simulink model "aircraft_6dof"  (R2025a)
settings: Solver=VariableStepAuto  StartTime=0.0  StopTime=sim_params.duration  FixedStep=0.01  RelTol=1e-8
undefined symbols (not defined in the file): aero, aircraft, atmos, control, controller, engine, IC
libraries: aerolibactuator x5, aerolibasang x2, aerolibfltsims x2, aerolibtransform2 x1, aerolibatmos2 x1, aerolibanimutils x1
settings Model: Creator=lordf  LastModifiedBy=lordf
settings DataIOCC: ExternalInput=getinputstruct(report1)  InitialState=getstatestruct(report1)

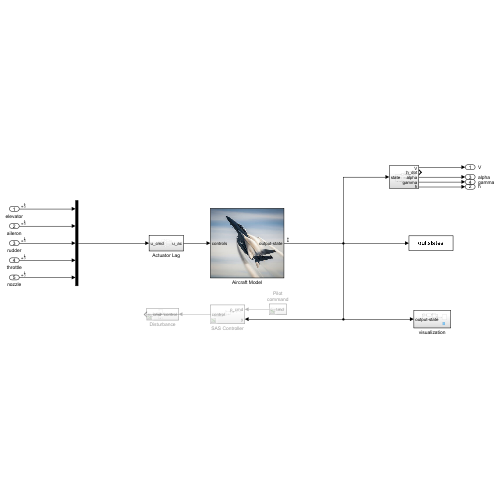
[thumbnail: Simulink's stored preview of the top-level diagram]
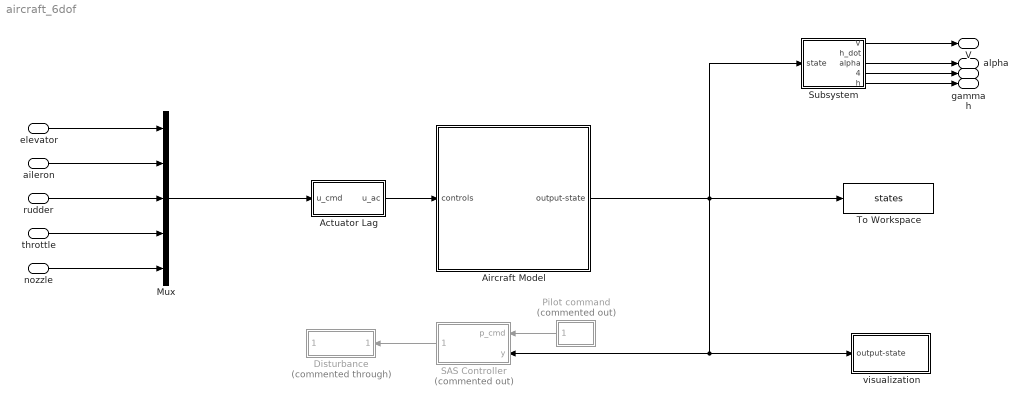
== system aircraft_6dof ==
  elevator : Inport
  aileron : Inport  Port=2
  rudder : Inport  Port=3
  throttle : Inport  Port=4
  nozzle : Inport  Port=5
  Actuator Lag : Subsystem
  Aircraft Model : Subsystem
      mask Display: image('Aircraft_image.jpg');
  Disturbance : Subsystem  Commented=through
  Mux : Mux  Inputs=5
  Pilot command : Subsystem  Commented=on
  SAS Controller : Subsystem  Commented=on
  Subsystem : Subsystem
  To Workspace : ToWorkspace  VariableName=states  SampleTime=-1
  visualization : Subsystem
  V : Outport
  h : Outport  Port=2
  alpha : Outport  Port=3
  gamma : Outport  Port=4
  wires:
  Subsystem/5(h) -> h/1
  Subsystem/1(V) -> V/1
  Subsystem/4(gamma) -> gamma/1
  Subsystem/3(alpha) -> alpha/1
  Actuator Lag/1(u_ac) -> Aircraft Model/1(controls)
  SAS Controller/1(control) -> Disturbance/1(control)
  Pilot command/1(p_cmd) -> SAS Controller/1(p_cmd)
  Aircraft Model/1(output-state) -> SAS Controller/2(y), visualization/1(output-state), Subsystem/1(state), To Workspace/1
  nozzle/1 -> Mux/5
  throttle/1 -> Mux/4
  aileron/1 -> Mux/2
  rudder/1 -> Mux/3
  elevator/1 -> Mux/1
  Mux/1 -> Actuator Lag/1(u_cmd)

== system aircraft_6dof/Actuator Lag ==
  u_cmd : Inport
  Demux : Demux  Outputs=5
  Mux : Mux  Inputs=5
  aileron lag : Subsystem
  elevator lag : Subsystem
  nozzle lag : Subsystem
  rudder lag : Subsystem
  throttle lag : Subsystem
  u_ac : Outport
  wires:
  u_cmd/1 -> Demux/1
  Mux/1 -> u_ac/1
  Demux/1 -> elevator lag/1(In1)
  elevator lag/1(Out1) -> Mux/1
  Demux/2 -> aileron lag/1(In1)
  aileron lag/1(Out1) -> Mux/2
  Demux/3 -> rudder lag/1(In1)
  rudder lag/1(Out1) -> Mux/3
  Demux/4 -> throttle lag/1(In1)
  throttle lag/1(Out1) -> Mux/4
  Demux/5 -> nozzle lag/1(In1)
  nozzle lag/1(Out1) -> Mux/5

== system aircraft_6dof/Aircraft Model ==
  controls : Inport
  6DOF (Euler Angles) : EOM6DOFBodyEuler  xme_0=[IC.x IC.y IC.z]  Vm_0=[IC.u, IC.v, IC.w]  eul_0=[IC.phi IC.theta IC.psi]  pm_0=[IC.p IC.q IC.r]  mass_0=aircraft.mass  inertia=aircraft.I
  Forces and Moments : Subsystem
  Mux1 : Mux
  output-state : Outport
  wires:
  6DOF (Euler Angles)/3 -> Mux1/4  "attitude(earth)"
  6DOF (Euler Angles)/5 -> Mux1/1  "velocity(body)"
  Forces and Moments/2(M) -> 6DOF (Euler Angles)/2
  6DOF (Euler Angles)/2 -> Mux1/2  "Position(earth)"
  Forces and Moments/1(F) -> 6DOF (Euler Angles)/1
  6DOF (Euler Angles)/6 -> Mux1/3  "omega(body)"
  controls/1 -> Forces and Moments/2(controls)
  Mux1/1 -> Forces and Moments/1(state), output-state/1

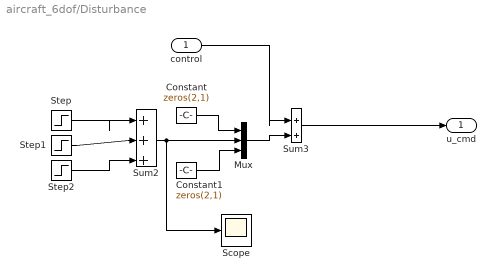
== system aircraft_6dof/Disturbance ==
  control : Inport
  Constant : Constant  Value=zeros(2,1)
  Constant1 : Constant  Value=zeros(2,1)
  Mux : Mux  Inputs=3
  Scope : Scope
      settings: ActiveDisplayYMinimum=-0.125  ActiveDisplayYMaximum=0.125
  Step : Step  Time=10  After=0.1  SampleTime=0
  Step1 : Step  Time=11  After=-0.2  SampleTime=0
  Step2 : Step  Time=12  After=0.1  SampleTime=0
  Sum2 : Sum  Inputs=|+++
  Sum3 : Sum  Inputs=|++
  u_cmd : Outport
  wires:
  Sum2/1 -> Mux/2, Scope/1
  Step/1 -> Sum2/1
  Step2/1 -> Sum2/3
  Step1/1 -> Sum2/2
  Sum3/1 -> u_cmd/1
  control/1 -> Sum3/1
  Mux/1 -> Sum3/2
  Constant/1 -> Mux/1
  Constant1/1 -> Mux/3

== system aircraft_6dof/Pilot command ==
  Gain : Gain  Gain=0.4
  Mux : Mux  Inputs=3
  Pilot Joystick : aerolibanimutils/Pilot Joystick  JoystickID=Joystick1  OutputConfiguration=FourAxis  SampleTime=1/30
  p_cmd : Outport
  wires:
  Mux/1 -> Gain/1
  Pilot Joystick/1 -> Mux/1
  Pilot Joystick/2 -> Mux/2
  Pilot Joystick/3 -> Mux/3
  Gain/1 -> p_cmd/1

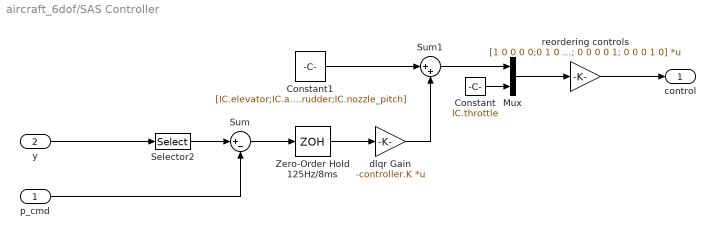
== system aircraft_6dof/SAS Controller ==
  p_cmd : Inport
  y : Inport  Port=2
  Constant : Constant  Value=IC.throttle
  Constant1 : Constant  Value=[IC.elevator;IC.aileron;IC.rudder;IC.nozzle_pitch]
  Mux : Mux  Inputs=2
  Selector2 : Selector  InputPortWidth=12  IndexOptions=Index vector (dialog)  Indices=7:9  OutputSizes=1
  Sum : Sum  Inputs=|+-
  Sum1 : Sum  Inputs=|++
  Zero-Order Hold 125Hz/8ms : ZeroOrderHold  SampleTime=controller.Ts
  dlqr Gain : Gain  Gain=-controller.K  Multiplication=Matrix(K*u)
  reordering controls : Gain  Gain=[1 0 0 0 0;0 1 0 0 0;0 0 1 0 0; 0 0 0 0 1; 0 0 0 1 0]  Multiplication=Matrix(K*u)
  control : Outport
  wires:
  Selector2/1 -> Sum/1
  y/1 -> Selector2/1
  Mux/1 -> reordering controls/1
  Constant1/1 -> Sum1/1
  Constant/1 -> Mux/2
  reordering controls/1 -> control/1
  Sum1/1 -> Mux/1
  dlqr Gain/1 -> Sum1/2
  Sum/1 -> Zero-Order Hold 125Hz/8ms/1
  p_cmd/1 -> Sum/2
  Zero-Order Hold 125Hz/8ms/1 -> dlqr Gain/1

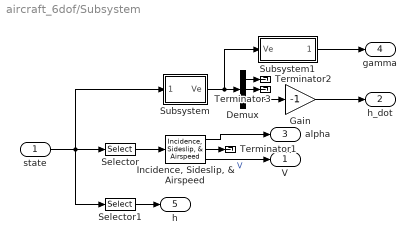
== system aircraft_6dof/Subsystem ==
  state : Inport
  Demux : Demux  Outputs=3
  Gain : Gain  Gain=-1
  "Incidence, Sideslip, & Airspeed" : aerolibasang/Incidence, Sideslip, & Airspeed
  Selector : Selector  InputPortWidth=12  IndexOptions=Index vector (dialog)  Indices=1:3  OutputSizes=1
  Selector1 : Selector  InputPortWidth=12  IndexOptions=Index vector (dialog)  Indices=6  OutputSizes=1
  Subsystem : Subsystem
  Subsystem1 : Subsystem
  Terminator1 : Terminator
  Terminator2 : Terminator
  Terminator3 : Terminator
  V : Outport
  h_dot : Outport  Port=2
  alpha : Outport  Port=3
  gamma : Outport  Port=4
  h : Outport  Port=5
  wires:
  Selector/1 -> "Incidence, Sideslip, & Airspeed"/1
  "Incidence, Sideslip, & Airspeed"/1 -> alpha/1
  "Incidence, Sideslip, & Airspeed"/2 -> Terminator1/1
  "Incidence, Sideslip, & Airspeed"/3 -> V/1  "V"
  Selector1/1 -> h/1
  state/1 -> Subsystem/1(state), Selector1/1, Selector/1
  Subsystem/1(Ve) -> Subsystem1/1(Ve), Demux/1
  Demux/3 -> Gain/1
  Demux/1 -> Terminator2/1
  Demux/2 -> Terminator3/1
  Gain/1 -> h_dot/1
  Subsystem1/1(gamma) -> gamma/1

== system aircraft_6dof/visualization ==
  output-state : Inport
  Constant : Constant  Value=-100
  Demux : Demux  Outputs=2
  Flat Earth to LLA : FlatEarth2LLA  LL0=[37.6655 -122.4809]
  FlightGear Preconfigured 6DoF Animation : aerolibfltsims/FlightGear Preconfigured 6DoF Animation  xFlightGearVersion=v2019.1  DestinationIpAddress=127.0.0.1  DestinationPort=5502  SampleTime=1/30  packetVersion=24
  Generate Run Script : aerolibfltsims/Generate Run Script  Architecture=Mac  dataFlow=Send  GeometryModelName=c172p  AirportId=KSFO  RunwayId=10L  InitialAltitude=7224  InitialHeading=113  OffsetDistance=4.72  OffsetAzimuth=0  InstallScenery=off  DisableShaders=off  OriginAddress=127.0.0.1  DestinationPort=5502  OriginPort=5505  LocalAddress=127.0.0.1  OutputFileName=runfg.bat  FlightGearBaseDirectory=C:\Program Files\FlightGear 2024.1
  Mux : Mux
  Selector : Selector  InputPortWidth=12  IndexOptions=Index vector (dialog)  Indices=10:12  OutputSizes=1
  Selector1 : Selector  InputPortWidth=12  IndexOptions=Index vector (dialog)  Indices=4:6  OutputSizes=1
  wires:
  output-state/1 -> Selector1/1, Selector/1
  Mux/1 -> FlightGear Preconfigured 6DoF Animation/1
  Selector/1 -> Mux/4
  Constant/1 -> Flat Earth to LLA/2
  Flat Earth to LLA/1 -> Demux/1
  Flat Earth to LLA/2 -> Mux/3
  Selector1/1 -> Flat Earth to LLA/1
  Demux/1 -> Mux/2
  Demux/2 -> Mux/1

== system aircraft_6dof/Actuator Lag/aileron lag ==
  In1 : Inport
  Linear Second-Order Actuator : aerolibactuator/Linear Second-Order Actuator  wn_fin=control.wn_aileron  z_fin=control.zeta_aileron  fin_act_0=IC.aileron  fin_act_vel=0
  Rate Limiter1 : RateLimiter  RisingSlewLimit=control.max_aileron_rate  FallingSlewLimit=-control.max_aileron_rate  SampleTimeMode=inherited
  Saturation1 : Saturate  UpperLimit=control.aileron_max  LowerLimit=-control.aileron_max
  Out1 : Outport
  wires:
  Linear Second-Order Actuator/1 -> Saturation1/1
  In1/1 -> Rate Limiter1/1
  Rate Limiter1/1 -> Linear Second-Order Actuator/1
  Saturation1/1 -> Out1/1

== system aircraft_6dof/Actuator Lag/elevator lag ==
  In1 : Inport
  Linear Second-Order Actuator : aerolibactuator/Linear Second-Order Actuator  wn_fin=control.wn_elevator  z_fin=control.zeta_elevator  fin_act_0=IC.elevator  fin_act_vel=0
  Rate Limiter : RateLimiter  RisingSlewLimit=control.max_elevator_rate  FallingSlewLimit=-control.max_elevator_rate  SampleTimeMode=inherited
  Saturation : Saturate  UpperLimit=control.elevator_max  LowerLimit=-control.elevator_max
  Out1 : Outport
  wires:
  In1/1 -> Rate Limiter/1
  Saturation/1 -> Out1/1
  Linear Second-Order Actuator/1 -> Saturation/1
  Rate Limiter/1 -> Linear Second-Order Actuator/1

== system aircraft_6dof/Actuator Lag/nozzle lag ==
  In1 : Inport
  Linear Second-Order Actuator : aerolibactuator/Linear Second-Order Actuator  wn_fin=control.wn_nozzle  z_fin=control.zeta_nozzle  fin_act_0=IC.nozzle_pitch  fin_act_vel=0
  Rate Limiter4 : RateLimiter  RisingSlewLimit=control.max_nozzle_rate  FallingSlewLimit=-control.max_nozzle_rate  SampleTimeMode=inherited
  Saturation4 : Saturate  UpperLimit=control.nozzle_pitch_max  LowerLimit=-control.nozzle_pitch_max
  Out1 : Outport
  wires:
  Rate Limiter4/1 -> Linear Second-Order Actuator/1
  Linear Second-Order Actuator/1 -> Saturation4/1
  Saturation4/1 -> Out1/1
  In1/1 -> Rate Limiter4/1

== system aircraft_6dof/Actuator Lag/rudder lag ==
  In1 : Inport
  Linear Second-Order Actuator : aerolibactuator/Linear Second-Order Actuator  wn_fin=control.wn_rudder  z_fin=control.zeta_rudder  fin_act_0=IC.rudder  fin_act_vel=0
  Rate Limiter2 : RateLimiter  RisingSlewLimit=control.max_rudder_rate  FallingSlewLimit=-control.max_rudder_rate  SampleTimeMode=inherited
  Saturation2 : Saturate  UpperLimit=control.rudder_max  LowerLimit=-control.rudder_max
  Out1 : Outport
  wires:
  Rate Limiter2/1 -> Linear Second-Order Actuator/1
  Linear Second-Order Actuator/1 -> Saturation2/1
  Saturation2/1 -> Out1/1
  In1/1 -> Rate Limiter2/1

== system aircraft_6dof/Actuator Lag/throttle lag ==
  In1 : Inport
  Linear Second-Order Actuator : aerolibactuator/Linear Second-Order Actuator  wn_fin=control.wn_throttle  z_fin=control.zeta_throttle  fin_act_0=IC.throttle  fin_act_vel=0
  Rate Limiter3 : RateLimiter  RisingSlewLimit=control.max_throttle_rate  FallingSlewLimit=-control.max_throttle_rate  SampleTimeMode=inherited
  Saturation3 : Saturate  UpperLimit=1  LowerLimit=0
  Out1 : Outport
  wires:
  Rate Limiter3/1 -> Linear Second-Order Actuator/1
  Saturation3/1 -> Out1/1
  Linear Second-Order Actuator/1 -> Saturation3/1
  In1/1 -> Rate Limiter3/1

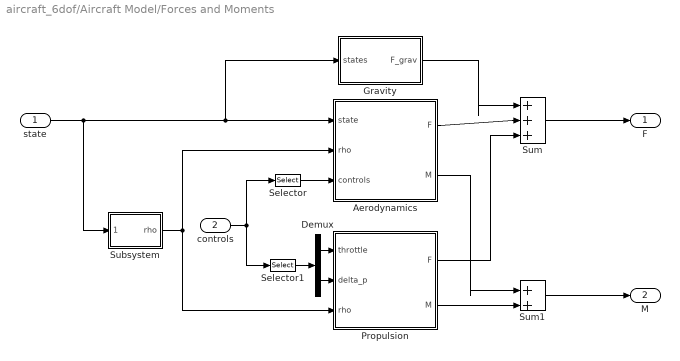
== system aircraft_6dof/Aircraft Model/Forces and Moments ==
  state : Inport
  controls : Inport  Port=2
  Aerodynamics : Subsystem
  Demux : Demux  Outputs=2
  Gravity : Subsystem
  Propulsion : Subsystem
  Selector : Selector  InputPortWidth=5  IndexOptions=Index vector (dialog)  Indices=1:3  OutputSizes=1
  Selector1 : Selector  InputPortWidth=5  IndexOptions=Index vector (dialog)  Indices=4:5  OutputSizes=1
  Subsystem : Subsystem
  Sum : Sum  Inputs=|+++
  Sum1 : Sum  Inputs=|++
  F : Outport
  M : Outport  Port=2
  wires:
  Sum/1 -> F/1
  Aerodynamics/1(F) -> Sum/2
  Aerodynamics/2(M) -> Sum1/1
  Gravity/1(F_grav) -> Sum/1
  Sum1/1 -> M/1
  Demux/1 -> Propulsion/1(throttle)
  Demux/2 -> Propulsion/2(delta_p)
  Propulsion/1(F) -> Sum/3
  Propulsion/2(M) -> Sum1/2
  Subsystem/1(rho) -> Aerodynamics/2(rho), Propulsion/3(rho)
  Selector/1 -> Aerodynamics/3(controls)
  Selector1/1 -> Demux/1
  controls/1 -> Selector1/1, Selector/1
  state/1 -> Subsystem/1(states), Aerodynamics/1(state), Gravity/1(states)

== system aircraft_6dof/Subsystem/Subsystem ==
  state : Inport
  Matrix Multiply : Product  Multiplication=Matrix(*)
  Rotation Angles to Direction Cosine Matrix : Angle2Dcm
      settings: AttributesFormatString=Rotation Order: %<rotationOrder>
  Selector : Selector  InputPortWidth=12  IndexOptions=Index vector (dialog)  Indices=10:12  OutputSizes=1
  Selector1 : Selector  InputPortWidth=12  IndexOptions=Index vector (dialog)  Indices=1:3  OutputSizes=1
  Transpose : Math  Operator=transpose
  Ve : Outport
  wires:
  Rotation Angles to Direction Cosine Matrix/1 -> Transpose/1
  state/1 -> Selector1/1, Selector/1
  Selector/1 -> Rotation Angles to Direction Cosine Matrix/1
  Transpose/1 -> Matrix Multiply/1
  Matrix Multiply/1 -> Ve/1
  Selector1/1 -> Matrix Multiply/2  "Vb"

== system aircraft_6dof/Subsystem/Subsystem1 ==
  Ve : Inport
  Atan2 : Trigonometry  Operator=atan2
  Demux : Demux  Outputs=3
  Gain1 : Gain  Gain=-1
  Square : Math  Operator=square
  Square Root : Sqrt
  Square1 : Math  Operator=square
  Sum : Sum  Inputs=|++
  gamma : Outport
  wires:
  Ve/1 -> Demux/1
  Gain1/1 -> Atan2/1
  Demux/3 -> Gain1/1
  Demux/2 -> Square1/1
  Demux/1 -> Square/1
  Square1/1 -> Sum/2
  Square/1 -> Sum/1
  Sum/1 -> Square Root/1
  Square Root/1 -> Atan2/2
  Atan2/1 -> gamma/1

== system aircraft_6dof/Aircraft Model/Forces and Moments/Aerodynamics ==
  state : Inport
  rho : Inport  Port=2
  controls : Inport  Port=3
  Aerodynamics : MATLAB Function  Commented=on  TreatAsAtomicUnit=on
  Forces : Subsystem
  "Incidence, Sideslip, & Airspeed" : aerolibasang/Incidence, Sideslip, & Airspeed
  Moments : Subsystem
  Selector : Selector  InputPortWidth=12  IndexOptions=Index vector (dialog)  Indices=1:3  OutputSizes=1
  Selector1 : Selector  InputPortWidth=12  IndexOptions=Index vector (dialog)  Indices=7:9  OutputSizes=1
  F : Outport
  M : Outport  Port=2
  wires:
  state/1 -> Selector/1, Selector1/1
  Moments/1(M) -> M/1
  Selector/1 -> "Incidence, Sideslip, & Airspeed"/1
  "Incidence, Sideslip, & Airspeed"/1 -> Forces/3(alpha), Moments/2(alpha)
  "Incidence, Sideslip, & Airspeed"/2 -> Forces/4(beta), Moments/1(beta)
  Forces/1(F) -> F/1
  "Incidence, Sideslip, & Airspeed"/3 -> Forces/5(V), Moments/3(V)  "V"
  rho/1 -> Forces/1(rho), Moments/4(rho)
  controls/1 -> Moments/5(controls), Forces/2(controls)
  Selector1/1 -> Moments/6(w_b)

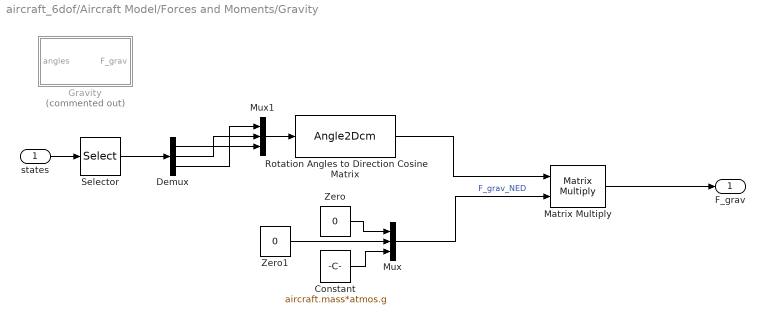
== system aircraft_6dof/Aircraft Model/Forces and Moments/Gravity ==
  states : Inport
  Constant : Constant  Value=aircraft.mass*atmos.g
  Demux : Demux  Outputs=3
  Gravity : MATLAB Function  Commented=on  TreatAsAtomicUnit=on
  Matrix Multiply : Product  Multiplication=Matrix(*)
  Mux : Mux  Inputs=3
  Mux1 : Mux  Inputs=3
  Rotation Angles to Direction Cosine Matrix : Angle2Dcm
      settings: AttributesFormatString=Rotation Order: %<rotationOrder>
  Selector : Selector  InputPortWidth=12  IndexOptions=Index vector (dialog)  Indices=10:12  OutputSizes=1
  Zero : Constant  Value=0  OutDataTypeStr=Inherit: Inherit via back propagation
  Zero1 : Constant  Value=0  OutDataTypeStr=Inherit: Inherit via back propagation
  F_grav : Outport
  wires:
  Matrix Multiply/1 -> F_grav/1
  states/1 -> Selector/1
  Selector/1 -> Demux/1
  Zero/1 -> Mux/1
  Zero1/1 -> Mux/2
  Constant/1 -> Mux/3
  Mux/1 -> Matrix Multiply/2  "F_grav_NED"
  Demux/2 -> Mux1/2
  Demux/1 -> Mux1/3
  Demux/3 -> Mux1/1
  Mux1/1 -> Rotation Angles to Direction Cosine Matrix/1
  Rotation Angles to Direction Cosine Matrix/1 -> Matrix Multiply/1

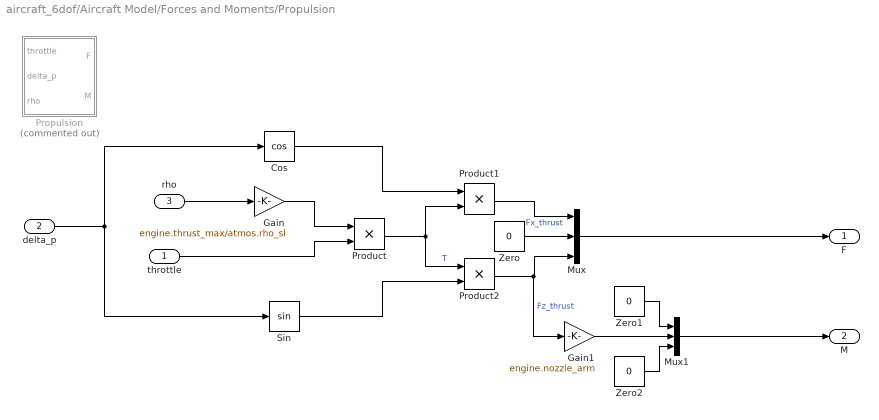
== system aircraft_6dof/Aircraft Model/Forces and Moments/Propulsion ==
  throttle : Inport
  delta_p : Inport  Port=2
  rho : Inport  Port=3
  Cos : Trigonometry  Operator=cos
  Gain : Gain  Gain=engine.thrust_max/atmos.rho_sl
  Gain1 : Gain  Gain=engine.nozzle_arm
  Mux : Mux  Inputs=3
  Mux1 : Mux  Inputs=3
  Product : Product
  Product1 : Product
  Product2 : Product
  Propulsion : MATLAB Function  Commented=on  TreatAsAtomicUnit=on
  Sin : Trigonometry
  Zero : Constant  Value=0  OutDataTypeStr=Inherit: Inherit via back propagation
  Zero1 : Constant  Value=0  OutDataTypeStr=Inherit: Inherit via back propagation
  Zero2 : Constant  Value=0  OutDataTypeStr=Inherit: Inherit via back propagation
  F : Outport
  M : Outport  Port=2
  wires:
  Gain1/1 -> Mux1/2
  delta_p/1 -> Sin/1, Cos/1
  rho/1 -> Gain/1
  Mux/1 -> F/1
  throttle/1 -> Product/2
  Gain/1 -> Product/1
  Product/1 -> Product2/1, Product1/2  "T"
  Cos/1 -> Product1/1
  Sin/1 -> Product2/2
  Product1/1 -> Mux/1  "Fx_thrust"
  Product2/1 -> Gain1/1, Mux/3  "Fz_thrust"
  Zero/1 -> Mux/2
  Mux1/1 -> M/1
  Zero1/1 -> Mux1/1
  Zero2/1 -> Mux1/3

== system aircraft_6dof/Aircraft Model/Forces and Moments/Subsystem ==
  states : Inport
  Gain : Gain  Gain=-1
  ISA Atmosphere Model : aerolibatmos2/ISA Atmosphere Model  useExtended=off  action=None  custom=off  viscosityOut=off  g=9.80665  gamma=1.4  R=287.0531  L=0.0065  h_trop=11000  h_strat=20000  rho0=1.225  P0=101325  T0=288.15  h0=0  S=110.4  Tref=273.15  muref=1.716e-5
  Selector : Selector  InputPortWidth=12  IndexOptions=Index vector (dialog)  Indices=6  OutputSizes=1
  rho : Outport
  wires:
  Selector/1 -> Gain/1
  Gain/1 -> ISA Atmosphere Model/1
  ISA Atmosphere Model/4 -> rho/1
  states/1 -> Selector/1

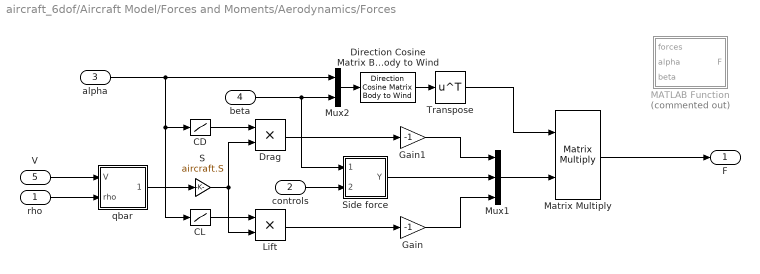
== system aircraft_6dof/Aircraft Model/Forces and Moments/Aerodynamics/Forces ==
  rho : Inport
  controls : Inport  Port=2
  alpha : Inport  Port=3
  beta : Inport  Port=4
  V : Inport  Port=5
  CD : Lookup_n-D  NumberOfTableDimensions=1  BreakpointsForDimension1=aero.alpha_table  Table=aero.CD_data  InterpMethod=Cubic spline  ExtrapMethod=Clip  InternalRulePriority=Speed  RndMeth=Simplest
  CL : Lookup_n-D  NumberOfTableDimensions=1  BreakpointsForDimension1=aero.alpha_table  Table=aero.CL_data  InterpMethod=Cubic spline  ExtrapMethod=Clip  InternalRulePriority=Speed  RndMeth=Simplest
  Direction Cosine Matrix Body to Wind : aerolibtransform2/Direction Cosine Matrix Body to Wind
  Drag : Product
  Gain : Gain  Gain=-1
  Gain1 : Gain  Gain=-1
  Lift : Product
  MATLAB Function : MATLAB Function  Commented=on  TreatAsAtomicUnit=on
  Matrix Multiply : Product  Multiplication=Matrix(*)
  Mux1 : Mux  Inputs=3
  Mux2 : Mux  Inputs=2
  S : Gain  Gain=aircraft.S
  Side force : Subsystem
  Transpose : Math  Operator=transpose
  qbar : Subsystem
  F : Outport
  wires:
  beta/1 -> Side force/1(Beta), Mux2/2
  qbar/1(qbar) -> S/1
  Drag/1 -> Gain1/1
  Mux1/1 -> Matrix Multiply/2
  Lift/1 -> Gain/1
  Gain1/1 -> Mux1/1
  Matrix Multiply/1 -> F/1
  Gain/1 -> Mux1/3
  CL/1 -> Lift/1
  Side force/1(Y) -> Mux1/2
  alpha/1 -> Mux2/1, CD/1, CL/1
  controls/1 -> Side force/2(controls)
  V/1 -> qbar/1(V)
  rho/1 -> qbar/2(rho)
  Direction Cosine Matrix Body to Wind/1 -> Transpose/1
  Transpose/1 -> Matrix Multiply/1
  Mux2/1 -> Direction Cosine Matrix Body to Wind/1
  CD/1 -> Drag/1
  S/1 -> Drag/2, Lift/2

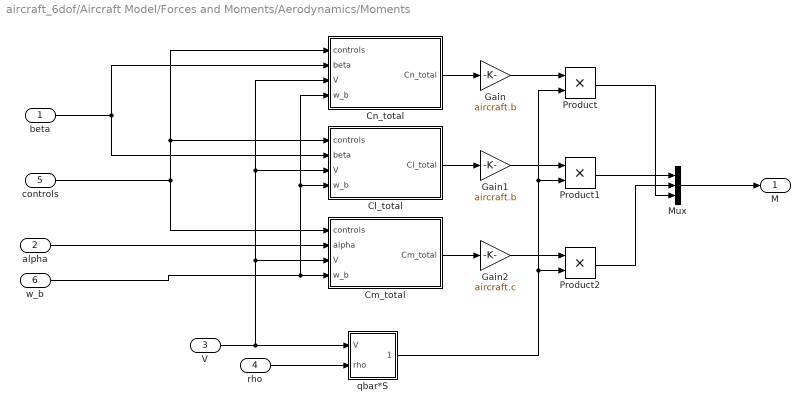
== system aircraft_6dof/Aircraft Model/Forces and Moments/Aerodynamics/Moments ==
  beta : Inport
  alpha : Inport  Port=2
  V : Inport  Port=3
  rho : Inport  Port=4
  controls : Inport  Port=5
  w_b : Inport  Port=6
  Cl_total : Subsystem
  Cm_total : Subsystem
  Cn_total : Subsystem
  Gain : Gain  Gain=aircraft.b
  Gain1 : Gain  Gain=aircraft.b
  Gain2 : Gain  Gain=aircraft.c
  Mux : Mux  Inputs=3
  Product : Product
  Product1 : Product
  Product2 : Product
  qbar*S : Subsystem
  M : Outport
  wires:
  rho/1 -> qbar*S/2(rho)
  V/1 -> qbar*S/1(V), Cn_total/3(V), Cl_total/3(V), Cm_total/3(V)
  qbar*S/1(qbar*S) -> Product2/2, Product1/2, Product/2
  alpha/1 -> Cm_total/2(alpha)
  Cm_total/1(Cm_total) -> Gain2/1
  controls/1 -> Cn_total/1(controls), Cl_total/1(controls), Cm_total/1(controls)
  w_b/1 -> Cn_total/4(w_b), Cl_total/4(w_b), Cm_total/4(w_b)
  beta/1 -> Cn_total/2(beta), Cl_total/2(beta)
  Mux/1 -> M/1
  Cl_total/1(Cl_total) -> Gain1/1
  Cn_total/1(Cn_total) -> Gain/1
  Gain/1 -> Product/1
  Gain1/1 -> Product1/1
  Gain2/1 -> Product2/1
  Product1/1 -> Mux/1
  Product2/1 -> Mux/2
  Product/1 -> Mux/3

== system aircraft_6dof/Aircraft Model/Forces and Moments/Aerodynamics/Forces/Side force ==
  Beta : Inport
  controls : Inport  Port=2
  Demux : Demux  Outputs=3
  Gain : Gain  Gain=aero.Cy_beta
  Gain1 : Gain  Gain=aero.Cy_dr
  Sum : Sum  Inputs=|++
  Y : Outport
  wires:
  Beta/1 -> Gain/1
  Gain/1 -> Sum/2
  Gain1/1 -> Sum/1
  Sum/1 -> Y/1
  controls/1 -> Demux/1
  Demux/3 -> Gain1/1

== system aircraft_6dof/Aircraft Model/Forces and Moments/Aerodynamics/Forces/qbar ==
  V : Inport
  rho : Inport  Port=2
  Gain : Gain  Gain=0.5
  Math Function : Math  Operator=square
  Product : Product
  qbar : Outport
  wires:
  Math Function/1 -> Product/1
  rho/1 -> Gain/1
  Gain/1 -> Product/2
  Product/1 -> qbar/1
  V/1 -> Math Function/1

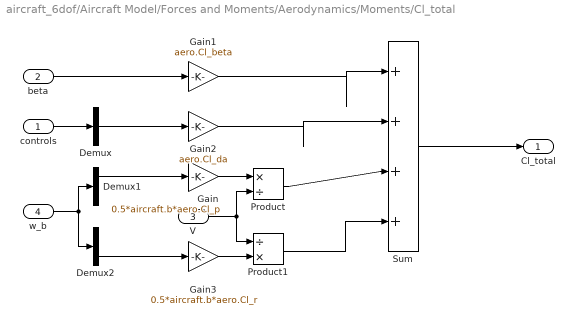
== system aircraft_6dof/Aircraft Model/Forces and Moments/Aerodynamics/Moments/Cl_total ==
  controls : Inport
  beta : Inport  Port=2
  V : Inport  Port=3
  w_b : Inport  Port=4
  Demux : Demux  Outputs=3
  Demux1 : Demux  Outputs=3
  Demux2 : Demux  Outputs=3
  Gain : Gain  Gain=0.5*aircraft.b*aero.Cl_p
  Gain1 : Gain  Gain=aero.Cl_beta
  Gain2 : Gain  Gain=aero.Cl_da
  Gain3 : Gain  Gain=0.5*aircraft.b*aero.Cl_r
  Product : Product  Inputs=*/
  Product1 : Product  Inputs=/*
  Sum : Sum  Inputs=|++++
  Cl_total : Outport
  wires:
  Sum/1 -> Cl_total/1
  Product/1 -> Sum/3
  controls/1 -> Demux/1
  V/1 -> Product/2, Product1/1
  Gain/1 -> Product/1
  w_b/1 -> Demux1/1, Demux2/1
  Gain1/1 -> Sum/1
  beta/1 -> Gain1/1
  Demux/2 -> Gain2/1
  Demux1/1 -> Gain/1
  Product1/1 -> Sum/4
  Gain3/1 -> Product1/2
  Demux2/3 -> Gain3/1
  Gain2/1 -> Sum/2

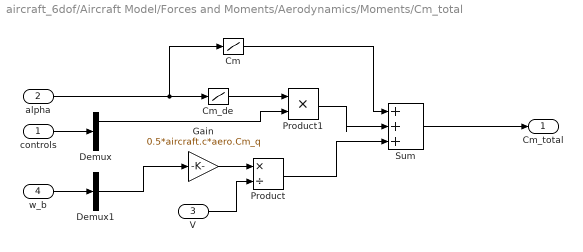
== system aircraft_6dof/Aircraft Model/Forces and Moments/Aerodynamics/Moments/Cm_total ==
  controls : Inport
  alpha : Inport  Port=2
  V : Inport  Port=3
  w_b : Inport  Port=4
  Cm : Lookup_n-D  NumberOfTableDimensions=1  BreakpointsForDimension1=aero.alpha_table  Table=aero.Cm_data  InterpMethod=Cubic spline  ExtrapMethod=Clip  InternalRulePriority=Speed  RndMeth=Simplest
  Cm_de : Lookup_n-D  NumberOfTableDimensions=1  BreakpointsForDimension1=aero.alpha_table  Table=aero.Cm_de_data  InterpMethod=Cubic spline  ExtrapMethod=Clip  InternalRulePriority=Speed  RndMeth=Simplest
  Demux : Demux  Outputs=3
  Demux1 : Demux  Outputs=3
  Gain : Gain  Gain=0.5*aircraft.c*aero.Cm_q
  Product : Product  Inputs=*/
  Product1 : Product
  Sum : Sum  Inputs=|+++
  Cm_total : Outport
  wires:
  alpha/1 -> Cm_de/1, Cm/1
  Cm_de/1 -> Product1/1
  Cm/1 -> Sum/1
  w_b/1 -> Demux1/1
  Gain/1 -> Product/1
  V/1 -> Product/2
  controls/1 -> Demux/1
  Demux/1 -> Product1/2
  Product1/1 -> Sum/2
  Product/1 -> Sum/3
  Sum/1 -> Cm_total/1
  Demux1/2 -> Gain/1

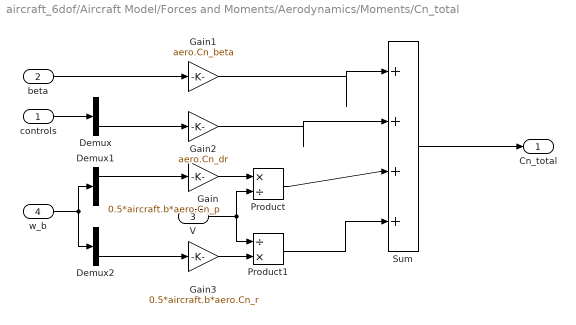
== system aircraft_6dof/Aircraft Model/Forces and Moments/Aerodynamics/Moments/Cn_total ==
  controls : Inport
  beta : Inport  Port=2
  V : Inport  Port=3
  w_b : Inport  Port=4
  Demux : Demux  Outputs=3
  Demux1 : Demux  Outputs=3
  Demux2 : Demux  Outputs=3
  Gain : Gain  Gain=0.5*aircraft.b*aero.Cn_p
  Gain1 : Gain  Gain=aero.Cn_beta
  Gain2 : Gain  Gain=aero.Cn_dr
  Gain3 : Gain  Gain=0.5*aircraft.b*aero.Cn_r
  Product : Product  Inputs=*/
  Product1 : Product  Inputs=/*
  Sum : Sum  Inputs=|++++
  Cn_total : Outport
  wires:
  Gain2/1 -> Sum/2
  Demux2/3 -> Gain3/1
  Gain3/1 -> Product1/2
  Product1/1 -> Sum/4
  Demux1/1 -> Gain/1
  Demux/3 -> Gain2/1
  beta/1 -> Gain1/1
  Gain1/1 -> Sum/1
  w_b/1 -> Demux2/1, Demux1/1
  Gain/1 -> Product/1
  V/1 -> Product1/1, Product/2
  controls/1 -> Demux/1
  Product/1 -> Sum/3
  Sum/1 -> Cn_total/1

== system aircraft_6dof/Aircraft Model/Forces and Moments/Aerodynamics/Moments/qbar*S ==
  V : Inport
  rho : Inport  Port=2
  Gain : Gain  Gain=0.5*aircraft.S
  Math Function : Math  Operator=square
  Product : Product
  qbar*S : Outport
  wires:
  V/1 -> Math Function/1
  Product/1 -> qbar*S/1
  Gain/1 -> Product/2
  rho/1 -> Gain/1
  Math Function/1 -> Product/1

== matlab function aircraft_6dof/Aircraft Model/Forces and Moments/Propulsion/Propulsion ==
  data: throttle input; F output; delta_p input; rho input; M output; engine parameter
function [F,M] = propulsion(throttle, delta_p, rho, engine)
% Forces and moments due to nozzle in body frame

rho_sl = 1.225;           % kg/m^3


% Thrust magnitude (altitude corrected)
sigma = rho / rho_sl;
T = engine.thrust_max * throttle * sigma;

% Forces in body frame
Fx_thrust = T * cos(delta_p);
Fy_thrust = 0.0;
Fz_thrust = T * sin(delta_p);

% Moment about CG
Mx_thrust = 0.0;
My_thrust = Fz_thrust * engine.nozzle_arm;
Mz_thrust = 0.0;

% Output
F = [Fx_thrust; Fy_thrust; Fz_thrust];
M = [Mx_thrust; My_thrust; Mz_thrust];
end

== matlab function aircraft_6dof/Aircraft Model/Forces and Moments/Aerodynamics/Aerodynamics ==
  data: state input; F output; controls input; rho input; M output; aero parameter; aircraft parameter
function [F,M]= aerodynamics(state, controls, rho, aero, aircraft)
% Aerodynamic forces and moments in body frame
% Unpack inputs
u = state(1); v = state(2); w = state(3);
p = state(4); q = state(5); r = state(6);
delta_e = controls(1); % elevator
delta_a = controls(2); % aileron
delta_r = controls(3); % rudder

% Flight parameters
V = sqrt(u^2+v^2+w^2);
if V<1e-6, V=1e-6; end
alpha = atan2(w,u);
beta = asin(v/V);

% Dynamic pressure
qbar = 0.5 * rho * V^2;

% Clamp alpha to table bounds
alpha_clamped = max(aero.alpha_min, min(alpha, aero.alpha_max));

% Interpolate aerodynamic coefficients using cubic spline
CL = interp1(aero.alpha_table, aero.CL_data, alpha_clamped, 'spline');
CD = interp1(aero.alpha_table, aero.CD_data, alpha_clamped, 'spline');
Cm = interp1(aero.alpha_table, aero.Cm_data, alpha_clamped, 'spline');
Cm_de = interp1(aero.alpha_table, aero.Cm_de_data, alpha_clamped, 'spline');

% Wind - frame forces
D = qbar * aircraft.S * CD; % Drag
L = qbar * aircraft.S * CL; % Lift
Y = qbar * aircraft.S * (aero.Cy_beta * beta + aero.Cy_dr * delta_r); % Side force

% Transform to body frame
ca = cos(alpha); sa = sin(alpha);
cb = cos(beta); sb = sin(beta);

% Aerodynamic forces
Fx_aero = -D * ca * cb - Y * sb + L * sa * cb;
Fy_aero = -D * ca * sb + Y * cb + L * sa * sb;
Fz_aero =  D * sa - L * ca;

% Aerodynamic moments
% Pitch Moment
Cm_total = Cm + aero.Cm_q*(q*aircraft.c/(2*V)) + Cm_de*delta_e;
My_aero = qbar * aircraft.S * aircraft.c * Cm_total;

% Roll Moment
Cl_beta_term = aero.Cl_beta * beta;
Cl_da_term   = aero.Cl_da * delta_a;
Cl_p_term    = aero.Cl_p * (p * aircraft.b / (2*V));
Cl_r_term    = aero.Cl_r * (r * aircraft.b / (2*V));
Mx_aero = qbar * aircraft.S * aircraft.b * (Cl_beta_term + Cl_da_term + Cl_p_term + Cl_r_term);

% Yaw Moment
Cn_beta_term = aero.Cn_beta * beta;
Cn_dr_term   = aero.Cn_dr * delta_r;
Cn_p_term    = aero.Cn_p * (p * aircraft.b / (2*V));
Cn_r_term    = aero.Cn_r * (r * aircraft.b / (2*V));
Mz_aero = qbar * aircraft.S * aircraft.b * (Cn_beta_term + Cn_dr_term + Cn_p_term + Cn_r_term);

% Output
F = [Fx_aero; Fy_aero; Fz_aero];
M = [Mx_aero; My_aero; Mz_aero];
end

== matlab function aircraft_6dof/Aircraft Model/Forces and Moments/Gravity/Gravity ==
  data: angles input; F_grav output; atmos parameter; aircraft parameter
function F_grav = gravity(angles, atmos, aircraft)
    % Gravity
    g = atmos.g;
    m = aircraft.mass;
    phi = angles(1);
    theta = angles(2);
    psi = angles(3);
    F_grav_ned = [0; 0; m*g];

    cphi = cos(phi); sphi = sin(phi);
    cth = cos(theta); sth = sin(theta);
    cpsi = cos(psi); spsi = sin(psi);
    
    C_bn = [cth*cpsi, cth*spsi, -sth;
            sphi*sth*cpsi - cphi*spsi, sphi*sth*spsi + cphi*cpsi, sphi*cth;
            cphi*sth*cpsi + sphi*spsi, cphi*sth*spsi - sphi*cpsi, cphi*cth];
    
    F_grav = C_bn * F_grav_ned;

end

== matlab function aircraft_6dof/Aircraft Model/Forces and Moments/Aerodynamics/Forces/MATLAB Function ==
  data: forces input; alpha input; F output; beta input
function F = fcn(forces,alpha,beta)
    % Transform to body frame
    ca = cos(alpha); sa = sin(alpha);
    cb = cos(beta);  sb = sin(beta);
    D = forces(1);
    Y = forces(2);
    L = forces(3);
    
    Fx_aero = -D * ca * cb - Y * sb + L * sa * cb;
    Fy_aero = -D * ca * sb + Y * cb + L * sa * sb;
    Fz_aero =  D * sa - L * ca;

    F = [Fx_aero;Fy_aero;Fz_aero];
